simulink model "SmAHTRHX_wcps"  (R2014a)
settings: Solver=ode3  StartTime=0.0  StopTime=400  FixedStep=.01  RelTol=1e-3
libraries: simulink x1
settings Model: Creator=LabUser  LastModifiedBy=wangwenchen
settings DebuggingCC: UnderspecifiedInitializationDetection=Classic  StateNameClashWarn=warning

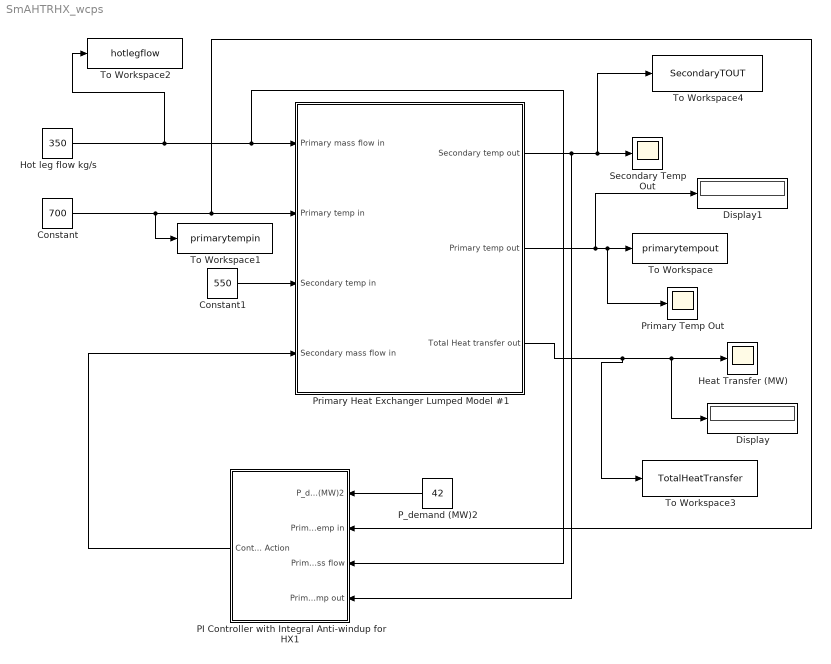
== system SmAHTRHX_wcps ==
  Constant : Constant  Value=700
  Constant1 : Constant  Value=550
  Display : Display
  Display1 : Display
  Heat Transfer (MW) : Scope
      settings: YMin=39  YMax=41.25  SaveName=ScopeData3
  Hot leg flow kg/s : Constant  Value=350
  PI Controller with Integral Anti-windup for HX1 : Subsystem
  P_demand (MW)2 : Constant  Value=42
  Primary Heat Exchanger Lumped Model #1 : Subsystem
  Primary Temp Out : Scope
      settings: SaveName=ScopeData2
  Secondary Temp Out : Scope
      settings: YMin=639  YMax=640.4
  To Workspace : ToWorkspace  VariableName=primarytempout  SaveFormat=Timeseries  SampleTime=-1
  To Workspace1 : ToWorkspace  VariableName=primarytempin  SaveFormat=Timeseries  SampleTime=-1
  To Workspace2 : ToWorkspace  VariableName=hotlegflow  SaveFormat=Timeseries  SampleTime=-1
  To Workspace3 : ToWorkspace  VariableName=TotalHeatTransfer  SaveFormat=Timeseries  SampleTime=-1
  To Workspace4 : ToWorkspace  VariableName=SecondaryTOUT  SaveFormat=Timeseries  SampleTime=-1
  wires:
  Primary Heat Exchanger Lumped Model #1/1(Secondary temp out) -> PI Controller with Integral Anti-windup for HX1/4(Primary temp out), To Workspace4/1, Secondary Temp Out/1
  Primary Heat Exchanger Lumped Model #1/2(Primary temp out) -> Display1/1, Primary Temp Out/1, To Workspace/1
  Constant/1 -> To Workspace1/1, PI Controller with Integral Anti-windup for HX1/2(Primary temp in), Primary Heat Exchanger Lumped Model #1/2(Primary temp in)
  Constant1/1 -> Primary Heat Exchanger Lumped Model #1/3(Secondary temp in)
  P_demand (MW)2/1 -> PI Controller with Integral Anti-windup for HX1/1(P_demand (MW)2)
  Hot leg flow kg/s/1 -> To Workspace2/1, PI Controller with Integral Anti-windup for HX1/3(Primary mass flow), Primary Heat Exchanger Lumped Model #1/1(Primary mass flow in)
  Primary Heat Exchanger Lumped Model #1/3("Total Heat transfer out ") -> To Workspace3/1, Display/1, Heat Transfer (MW)/1
  PI Controller with Integral Anti-windup for HX1/1(Control Action) -> Primary Heat Exchanger Lumped Model #1/4(Secondary mass flow in)

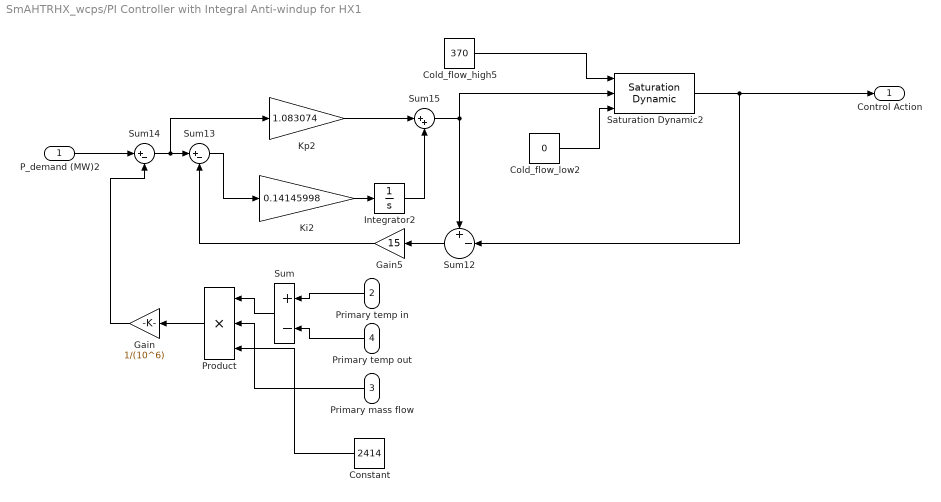
== system SmAHTRHX_wcps/PI Controller with Integral Anti-windup for HX1 ==
  P_demand (MW)2 : Inport
  Primary temp in : Inport  Port=2
  Primary mass flow : Inport  Port=3
  Primary temp out : Inport  Port=4
  Cold_flow_high5 : Constant  Value=370
  Cold_flow_low2 : Constant  Value=0
  Constant : Constant  Value=2414
  Gain : Gain  Gain=1/(10^6)
  Gain5 : Gain  Gain=15
  Integrator2 : Integrator  InitialCondition=100
  Ki2 : Gain  Gain=0.14145998
  Kp2 : Gain  Gain=1.083074
  Product : Product  Inputs=3
  Saturation Dynamic2 : simulink/Discontinuities/Saturation Dynamic  OutMin=[]  OutMax=[]  OutDataTypeStr=Inherit: Same as second input  OutDataType=fixdt(1, 16)  OutScaling=2^-10  DoSatur=off
  Sum : Sum  Inputs=+-
  Sum12 : Sum  Inputs=+-|
  Sum13 : Sum  Inputs=|+-
  Sum14 : Sum  Inputs=|+-
  Sum15 : Sum  Inputs=|++
  Control Action : Outport
  wires:
  Product/1 -> Gain/1
  Cold_flow_low2/1 -> Saturation Dynamic2/3
  Cold_flow_high5/1 -> Saturation Dynamic2/1
  Sum14/1 -> Kp2/1, Sum13/1
  P_demand (MW)2/1 -> Sum14/1
  Sum12/1 -> Gain5/1
  Integrator2/1 -> Sum15/2
  Gain5/1 -> Sum13/2
  Sum13/1 -> Ki2/1
  Ki2/1 -> Integrator2/1
  Kp2/1 -> Sum15/1
  Saturation Dynamic2/1 -> Control Action/1, Sum12/2
  Sum15/1 -> Sum12/1, Saturation Dynamic2/2
  Primary temp in/1 -> Sum/1
  Primary temp out/1 -> Sum/2
  Sum/1 -> Product/1
  Primary mass flow/1 -> Product/2
  Constant/1 -> Product/3
  Gain/1 -> Sum14/2

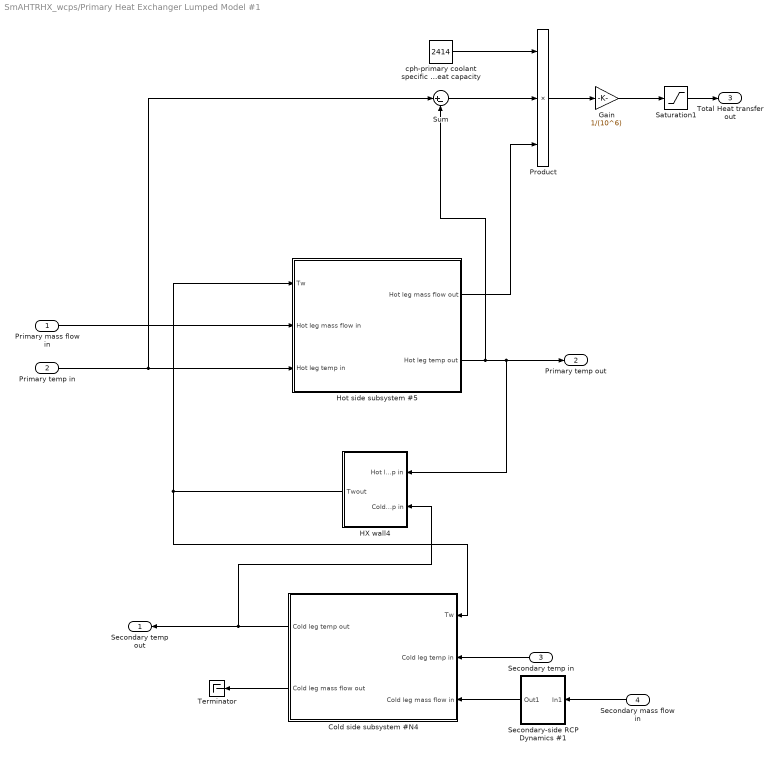
== system SmAHTRHX_wcps/Primary Heat Exchanger Lumped Model #1 ==
  Primary mass flow in : Inport
  Primary temp in : Inport  Port=2
  Secondary temp in : Inport  Port=3
  Secondary mass flow in : Inport  Port=4
  Cold side subsystem #N4 : Subsystem
  Gain : Gain  Gain=1/(10^6)
  HX wall4 : Subsystem
  Hot side subsystem #5 : Subsystem
  Product : Product  Inputs=3
  Saturation1 : Saturate  UpperLimit=inf  LowerLimit=0
  Secondary-side RCP Dynamics #1 : Subsystem
  Sum : Sum  Inputs=|+-
  Terminator : Terminator
  cph-primary coolant specific heat capacity : Constant  Value=2414
  Secondary temp out : Outport
  Primary temp out : Outport  Port=2
  "Total Heat transfer out " : Outport  Port=3
  wires:
  Cold side subsystem #N4/1(Cold leg temp out) -> Secondary temp out/1, HX wall4/2(Cold leg temp in)
  Cold side subsystem #N4/2(Cold leg mass flow out) -> Terminator/1
  Primary mass flow in/1 -> Hot side subsystem #5/2(Hot leg mass flow in)
  Primary temp in/1 -> Hot side subsystem #5/3(Hot leg temp in), Sum/1
  Secondary mass flow in/1 -> Secondary-side RCP Dynamics #1/1(In1)
  Secondary temp in/1 -> Cold side subsystem #N4/2(Cold leg temp in)
  HX wall4/1(Twout) -> Cold side subsystem #N4/1(Tw), Hot side subsystem #5/1(Tw)
  Hot side subsystem #5/1(Hot leg mass flow out) -> Product/3
  Hot side subsystem #5/2(Hot leg temp out) -> HX wall4/1(Hot leg temp in), Primary temp out/1, Sum/2
  cph-primary coolant specific heat capacity/1 -> Product/1
  Sum/1 -> Product/2
  Product/1 -> Gain/1
  Gain/1 -> Saturation1/1
  Secondary-side RCP Dynamics #1/1(Out1) -> Cold side subsystem #N4/3(Cold leg mass flow in)
  Saturation1/1 -> "Total Heat transfer out "/1

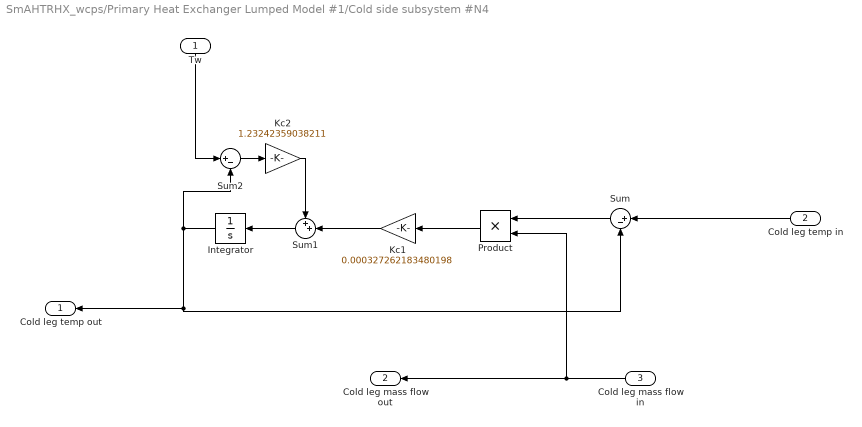
== system SmAHTRHX_wcps/Primary Heat Exchanger Lumped Model #1/Cold side subsystem #N4 ==
  Tw : Inport
  Cold leg temp in : Inport  Port=2
  Cold leg mass flow in : Inport  Port=3
  Integrator : Integrator  InitialCondition=600
  Kc1 : Gain  Gain=0.000327262183480198
  Kc2 : Gain  Gain=1.23242359038211
  Product : Product
  Sum : Sum  Inputs=|+-
  Sum1 : Sum  Inputs=++|
  Sum2 : Sum  Inputs=|+-
  Cold leg temp out : Outport
  Cold leg mass flow out : Outport  Port=2
  wires:
  Cold leg temp in/1 -> Sum/1
  Integrator/1 -> Sum/2, Cold leg temp out/1, Sum2/2
  Sum2/1 -> Kc2/1
  Sum/1 -> Product/1
  Kc2/1 -> Sum1/1
  Sum1/1 -> Integrator/1
  Cold leg mass flow in/1 -> Cold leg mass flow out/1, Product/2
  Product/1 -> Kc1/1
  Kc1/1 -> Sum1/2
  Tw/1 -> Sum2/1

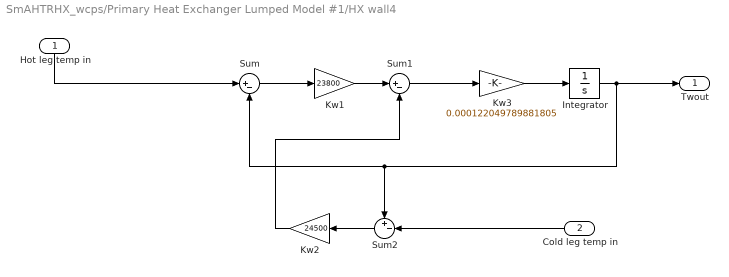
== system SmAHTRHX_wcps/Primary Heat Exchanger Lumped Model #1/HX wall4 ==
  Hot leg temp in : Inport
  Cold leg temp in : Inport  Port=2
  Integrator : Integrator  InitialCondition=650
  Kw1 : Gain  Gain=23800
  Kw2 : Gain  Gain=24500
  Kw3 : Gain  Gain=0.000122049789881805
  Sum : Sum  Inputs=|+-
  Sum1 : Sum  Inputs=|+-
  Sum2 : Sum  Inputs=+-|
  Twout : Outport
  wires:
  Sum2/1 -> Kw2/1
  Hot leg temp in/1 -> Sum/1
  Sum1/1 -> Kw3/1
  Cold leg temp in/1 -> Sum2/2
  Sum/1 -> Kw1/1
  Kw1/1 -> Sum1/1
  Kw3/1 -> Integrator/1
  Integrator/1 -> Twout/1, Sum2/1, Sum/2
  Kw2/1 -> Sum1/2

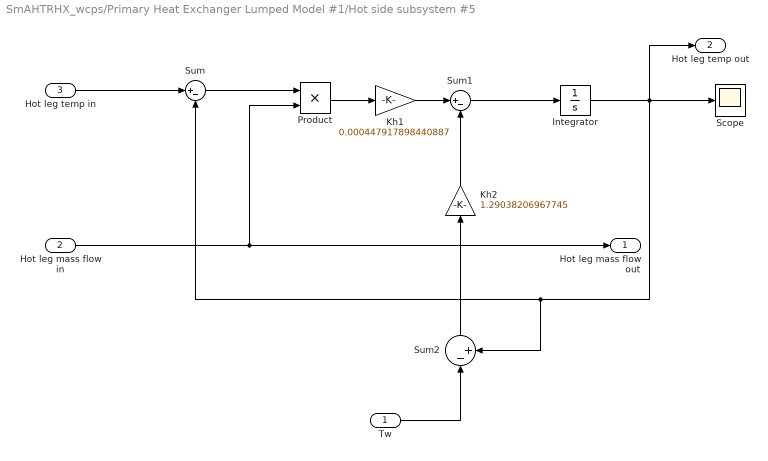
== system SmAHTRHX_wcps/Primary Heat Exchanger Lumped Model #1/Hot side subsystem #5 ==
  Tw : Inport
  Hot leg mass flow in : Inport  Port=2
  Hot leg temp in : Inport  Port=3
  Integrator : Integrator  InitialCondition=700
  Kh1 : Gain  Gain=0.000447917898440887
  Kh2 : Gain  Gain=1.29038206967745
  Product : Product
  Scope : Scope
  Sum : Sum  Inputs=|+-
  Sum1 : Sum  Inputs=|+-
  Sum2 : Sum  Inputs=|-+
  Hot leg mass flow out : Outport
  Hot leg temp out : Outport  Port=2
  wires:
  Product/1 -> Kh1/1
  Kh1/1 -> Sum1/1
  Sum1/1 -> Integrator/1
  Sum2/1 -> Kh2/1
  Kh2/1 -> Sum1/2
  Tw/1 -> Sum2/1
  Hot leg temp in/1 -> Sum/1
  Hot leg mass flow in/1 -> Hot leg mass flow out/1, Product/2
  Sum/1 -> Product/1
  Integrator/1 -> Hot leg temp out/1, Scope/1, Sum2/2, Sum/2

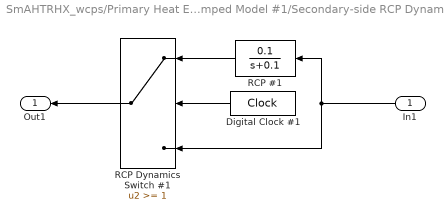
== system SmAHTRHX_wcps/Primary Heat Exchanger Lumped Model #1/Secondary-side RCP Dynamics #1 ==
  In1 : Inport
  Digital Clock #1 : DigitalClock  SampleTime=.01
  RCP #1 : TransferFcn  Numerator=[0.1]  Denominator=[1 0.1]
  RCP Dynamics Switch #1 : Switch  Threshold=1
  Out1 : Outport
  wires:
  In1/1 -> RCP #1/1, RCP Dynamics Switch #1/3
  Digital Clock #1/1 -> RCP Dynamics Switch #1/2
  RCP #1/1 -> RCP Dynamics Switch #1/1
  RCP Dynamics Switch #1/1 -> Out1/1
